simulink model "TPG"  (R2018b)
settings: Solver=VariableStepAuto  StartTime=0.0  StopTime=10.0  RelTol=1e-3
values from neighbouring files (symbols this model uses):
  ts = 1/1000    (= 0.001)    [Tflex_Controller_init.m]
undefined symbols (not defined in the file or in its folder): DiscIntNeverNeededParam, h, r
settings Model: Creator=Dave Vogel  LastModifiedBy=Dave Vogel

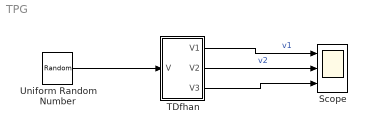
== system TPG ==
  Scope : Scope  NumInputPorts=3
  TDfhan : Subsystem
  Uniform Random Number : UniformRandomNumber  Minimum=-25  Maximum=25  SampleTime=0.5
  wires:
  Uniform Random Number/1 -> TDfhan/1(V)
  TDfhan/2(V2) -> Scope/2  "v2"
  TDfhan/1(V1) -> Scope/1  "v1"
  TDfhan/3(V3) -> Scope/3

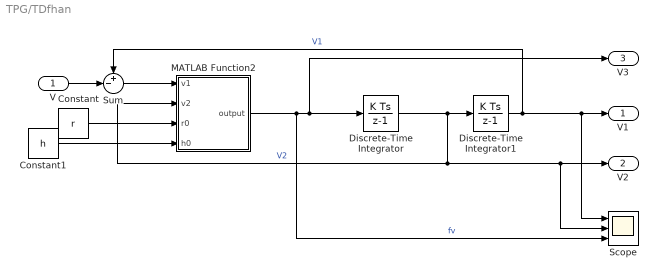
== system TPG/TDfhan ==
  V : Inport
  Constant : Constant  Value=r
  Constant1 : Constant  Value=h
  Discrete-Time Integrator : DiscreteIntegrator  gainval=1  SampleTime=ts  ICPrevOutput=DiscIntNeverNeededParam  ICPrevScaledInput=DiscIntNeverNeededParam
  Discrete-Time Integrator1 : DiscreteIntegrator  gainval=1  SampleTime=ts  ICPrevOutput=DiscIntNeverNeededParam  ICPrevScaledInput=DiscIntNeverNeededParam
  MATLAB Function2 : MATLAB Function  TreatAsAtomicUnit=on
  Scope : Scope  NumInputPorts=3
  Sum : Sum  Inputs=+-|
  V1 : Outport
  V2 : Outport  Port=2
  V3 : Outport  Port=3
  wires:
  Discrete-Time Integrator/1 -> Discrete-Time Integrator1/1, MATLAB Function2/2(v2), Scope/2, V2/1  "V2"
  Discrete-Time Integrator1/1 -> Scope/1, V1/1, Sum/1  "V1"
  MATLAB Function2/1(output) -> Scope/3, V3/1, Discrete-Time Integrator/1  "fv"
  Sum/1 -> MATLAB Function2/1(v1)
  V/1 -> Sum/2
  Constant/1 -> MATLAB Function2/3(r0)
  Constant1/1 -> MATLAB Function2/4(h0)

== matlab function TPG/TDfhan/MATLAB Function2 ==
  data: v1 input; output output; v2 input; r0 input; h0 input
function output = Fhan(v1,v2,r0, h0)
d = h0^2*r0;
a0 = h0*v2;
y = v1 + a0;
a1 = sqrt(d*(d+8*abs(y)));
a2 = a0 + sign(y)*(a1-d)/2;
sy = (sign(y+d)-sign(y-d))/2;
a = (a0+y-a2)*sy +a2;
sa = (sign(a+d)-sign(a-d))/2;
output = -r0 *(a/d -sign(a) )*sa - r0*sign(a);
